simulink model "control_system"  (R2024a)
settings: Solver=VariableStepAuto  StartTime=0.0  StopTime=10.0  RelTol=1e-3
undefined symbols (not defined in the file): a, Cvx1, Cvx2, Cwy1, Cwy2, Jy, K, k, K1_k, K1_m, K2, K2_m, L11, L55, m, Mb, T, Umax, V_streem
libraries: dspsnks4 x1
settings Model: Creator=gbogu  LastModifiedBy=mikle
settings RTWCC: GPUComputeCapability=3.5

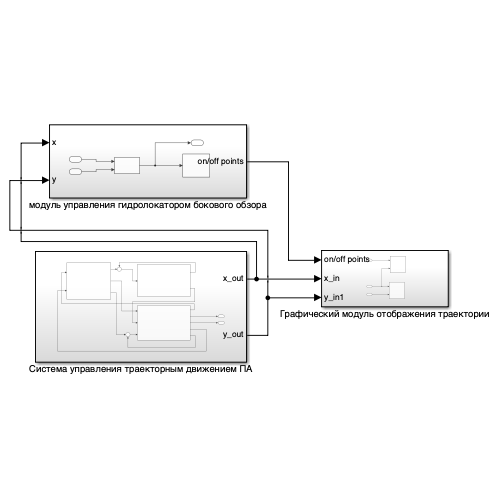
[thumbnail: Simulink's stored preview of the top-level diagram]
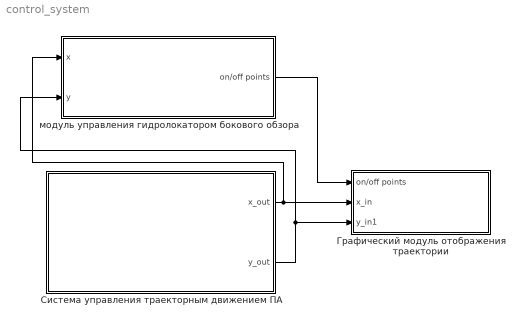
== system control_system ==
  Графический модуль отображения траектории : Subsystem
  Система управления траекторным движением ПА : Subsystem
  модуль управления гидролокатором бокового обзора : Subsystem
  wires:
  Система управления траекторным движением ПА/1(x_out) -> модуль управления гидролокатором бокового обзора/1(x), Графический модуль отображения траектории/2(x_in)
  Система управления траекторным движением ПА/2(y_out) -> модуль управления гидролокатором бокового обзора/2(y), Графический модуль отображения траектории/3(y_in1)
  модуль управления гидролокатором бокового обзора/1(on/off points) -> Графический модуль отображения траектории/1(on/off points)

== system control_system/Графический модуль отображения траектории ==
  on/off points : Inport
  x_in : Inport  Port=2
  y_in1 : Inport  Port=3
  XY Graph : Record  FileSettingsInternal="{\"entries\":[{\"content\":{\"excelSettings\":{\"content\":{},\"type\":\"Streamout.ExcelSettings\"}},\"type\":\"Streamout.FileSettingStorage\",\"uuid\":\"\"}],\"packageUris\":[\"http:\\/\\/schema.mathworks.com\\/mf0\\/streamout_blocks\\/R2020a\"],\"version\":\"1.0\"}"  Layout=[1 1]  SignalsInternal="{\"entries\":[{\"content\":{\"signals\":[{\"content\":{\"blockPath\":[],\"dimensions\":[1],\"domain\":\"\",\"lineColor\":\"#a2142f\",\"plots\":[ 1 ],\"port\":1,\"signalID\":1,\"signalName\":\"XY Graph:1\"},\"type\":\"RecordBlkView.Signal\",\"uuid\":\"\"},{\"content\":{\"blockPath\":[],\"dimensions\":[1],\"domain\":\"\",\"lineColor\":\"#139fff\",\"plots\":[ 1 ],\"port\":2,\"signalID\":2,\"signalName\":\"XY Graph:2\"},\"type\":\"RecordBlkView.Signal\",\"uuid\":\"\"}]},\"type\":\"RecordBlkView.InputSignals\",\"uuid\":\"\"}],\"packageUris\":[\"http:\\/\\/schema.mathworks.com\\/mf0\\/streamout_blocks\\/R2020a\"],\"version\":\"1.0\"}"  VisualizationBindings="{\"xyplotplugin\":{\"info\":[{\"series\":[{\"bindingParametersList\":[{\"parameter\":\"X-Axis\",\"signalID\":1,\"signalName\":\"XY Graph:1\"},{\"parameter\":\"Y-Axis\",\"signalID\":2,\"signalName\":\"XY Graph:2\"}],\"seriesID\":0}],\"subplotID\":1}]}}"  CompatibilityTag=XY
  XY Graph1 : Record  FileSettingsInternal="{\"entries\":[{\"content\":{\"excelSettings\":{\"content\":{},\"type\":\"Streamout.ExcelSettings\"}},\"type\":\"Streamout.FileSettingStorage\",\"uuid\":\"\"}],\"packageUris\":[\"http:\\/\\/schema.mathworks.com\\/mf0\\/streamout_blocks\\/R2020a\"],\"version\":\"1.0\"}"  Layout=[1 1]  SignalsInternal="{\"entries\":[{\"content\":{\"signals\":[{\"content\":{\"blockPath\":[],\"dimensions\":[1],\"domain\":\"\",\"lineColor\":\"#a2142f\",\"plots\":[ 1 ],\"port\":1,\"signalID\":1,\"signalName\":\"XY Graph:1\"},\"type\":\"RecordBlkView.Signal\",\"uuid\":\"\"},{\"content\":{\"blockPath\":[],\"dimensions\":[1],\"domain\":\"\",\"lineColor\":\"#139fff\",\"plots\":[ 1 ],\"port\":2,\"signalID\":2,\"signalName\":\"XY Graph:2\"},\"type\":\"RecordBlkView.Signal\",\"uuid\":\"\"}]},\"type\":\"RecordBlkView.InputSignals\",\"uuid\":\"\"}],\"packageUris\":[\"http:\\/\\/schema.mathworks.com\\/mf0\\/streamout_blocks\\/R2020a\"],\"version\":\"1.0\"}"  VisualizationBindings="{\"xyplotplugin\":{\"info\":[{\"series\":[{\"bindingParametersList\":[{\"parameter\":\"X-Axis\",\"signalID\":1,\"signalName\":\"XY Graph:1\"},{\"parameter\":\"Y-Axis\",\"signalID\":2,\"signalName\":\"XY Graph:2\"}],\"seriesID\":0}],\"subplotID\":1}]}}"  CompatibilityTag=XY
  wires:
  y_in1/1 -> XY Graph/2  "y"
  x_in/1 -> XY Graph1/2, XY Graph/1  "r_in"
  on/off points/1 -> XY Graph1/1

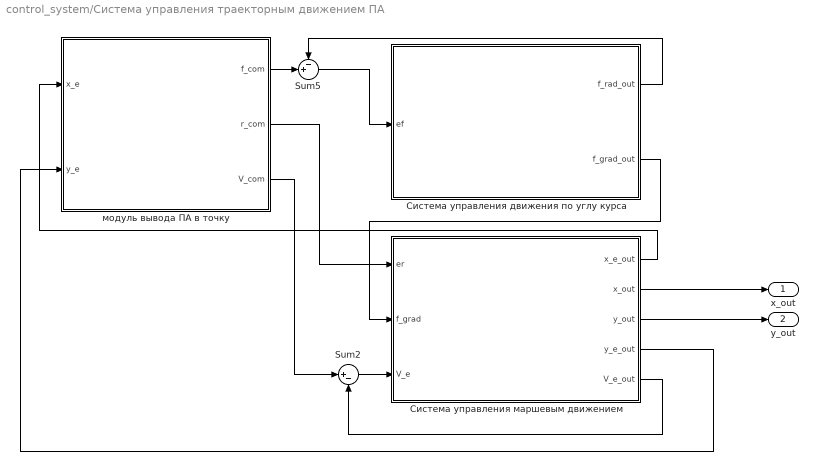
== system control_system/Система управления траекторным движением ПА ==
  Sum2 : Sum  Inputs=|+-
  Sum5 : Sum  Inputs=-+|
  "Система управления движения по углу курса " : Subsystem
  Система управления маршевым движением : Subsystem
  модуль вывода ПА в точку : Subsystem
  x_out : Outport
  y_out : Outport  Port=2
  wires:
  модуль вывода ПА в точку/1(f_com) -> Sum5/2
  модуль вывода ПА в точку/3(V_com) -> Sum2/1
  модуль вывода ПА в точку/2(r_com) -> Система управления маршевым движением/1(er)
  Sum2/1 -> Система управления маршевым движением/3(V_e)
  Система управления маршевым движением/1(x_e_out) -> модуль вывода ПА в точку/1(x_e)
  Система управления маршевым движением/2(x_out) -> x_out/1
  Система управления маршевым движением/3(y_out) -> y_out/1
  Система управления маршевым движением/4(y_e_out) -> модуль вывода ПА в точку/2(y_e)
  Система управления маршевым движением/5(V_e_out) -> Sum2/2
  "Система управления движения по углу курса "/2(f_grad_out) -> Система управления маршевым движением/2(f_grad)
  Sum5/1 -> "Система управления движения по углу курса "/1(ef)
  "Система управления движения по углу курса "/1(f_rad_out) -> Sum5/1

== system control_system/модуль управления гидролокатором бокового обзора ==
  x : Inport
  y : Inport  Port=2
  Function Caller : FunctionCaller  FunctionPrototype=y = f(x,y)  InputArgumentSpecifications=<Enter example>  OutputArgumentSpecifications=<Enter example>
  гидролокатор бокового обзора : dspsnks4/Audio Device Writer  Driver=CoreAudio  Device=Default  InheritSampleRate=on  SampleRate=44100  BitDepth=16-bit integer  BufferSize=4096  NumBuffers=10  DefaultOutputChannelMapping=on  OutputChannelMapping=1:2  OutputNumUnderrunSamples=off  DriverIdx=5  DeviceWarnFlag=''
  on/off points : Outport
  wires:
  x/1 -> Function Caller/1
  y/1 -> Function Caller/2
  Function Caller/1 -> on/off points/1, гидролокатор бокового обзора/1

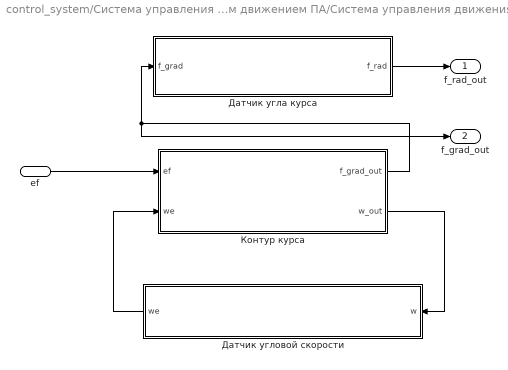
== system control_system/Система управления траекторным движением ПА/Система управления движения по углу курса  ==
  ef : Inport
  Датчик угла курса : Subsystem
  Датчик угловой скорости : Subsystem
  Контур курса : Subsystem
  f_rad_out : Outport
  f_grad_out : Outport  Port=2
  wires:
  ef/1 -> Контур курса/1(ef)
  Контур курса/2(w_out) -> Датчик угловой скорости/1(w)
  Контур курса/1(f_grad_out) -> f_grad_out/1, Датчик угла курса/1(f_grad)
  Датчик угла курса/1(f_rad) -> f_rad_out/1
  Датчик угловой скорости/1(we) -> Контур курса/2(we)

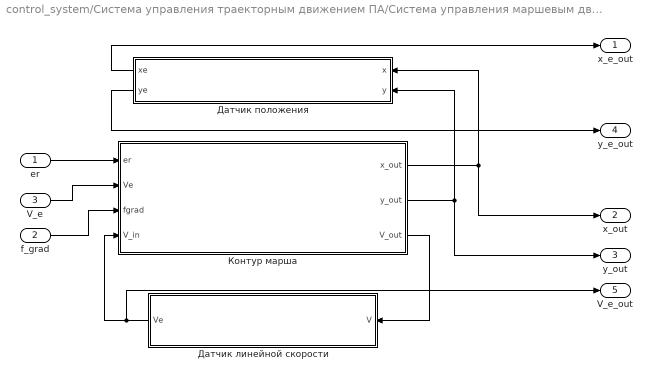
== system control_system/Система управления траекторным движением ПА/Система управления маршевым движением ==
  er : Inport
  f_grad : Inport  Port=2
  V_e : Inport  Port=3
  Датчик линейной скорости : Subsystem
  Датчик положения : Subsystem
  Контур марша : Subsystem
  x_e_out : Outport
  x_out : Outport  Port=2
  y_out : Outport  Port=3
  y_e_out : Outport  Port=4
  V_e_out : Outport  Port=5
  wires:
  er/1 -> Контур марша/1(er)
  Датчик положения/2(ye) -> y_e_out/1
  Датчик положения/1(xe) -> x_e_out/1
  Контур марша/3(V_out) -> Датчик линейной скорости/1(V)
  V_e/1 -> Контур марша/2(Ve)
  Контур марша/1(x_out) -> Датчик положения/1(x), x_out/1
  Контур марша/2(y_out) -> Датчик положения/2(y), y_out/1
  f_grad/1 -> Контур марша/3(fgrad)
  Датчик линейной скорости/1(Ve) -> Контур марша/4(V_in), V_e_out/1

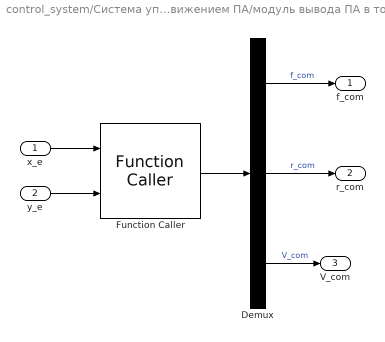
== system control_system/Система управления траекторным движением ПА/модуль вывода ПА в точку ==
  x_e : Inport
  y_e : Inport  Port=2
  Demux : Demux  Outputs=3
  Function Caller : FunctionCaller  FunctionPrototype=Vel = f(x_e,y_e)  InputArgumentSpecifications=<Enter example>  OutputArgumentSpecifications=<Enter example>
  f_com : Outport
  r_com : Outport  Port=2
  V_com : Outport  Port=3
  wires:
  Demux/3 -> V_com/1  "V_com"
  Demux/1 -> f_com/1  "f_com"
  Demux/2 -> r_com/1  "r_com"
  y_e/1 -> Function Caller/2
  x_e/1 -> Function Caller/1
  Function Caller/1 -> Demux/1

== system control_system/Система управления траекторным движением ПА/Система управления движения по углу курса /Датчик угла курса ==
  f_grad : Inport
  Gain10 : Gain  Gain=pi/180
  angle sensore : Gain  Gain=93.1395
  f_rad : Outport
  wires:
  Gain10/1 -> f_rad/1  "frad"
  f_grad/1 -> angle sensore/1
  angle sensore/1 -> Gain10/1  "fe"

== system control_system/Система управления траекторным движением ПА/Система управления движения по углу курса /Датчик угловой скорости ==
  w : Inport
  omega sensor : Gain  Gain=93.1395
  we : Outport
  wires:
  omega sensor/1 -> we/1  "we"
  w/1 -> omega sensor/1

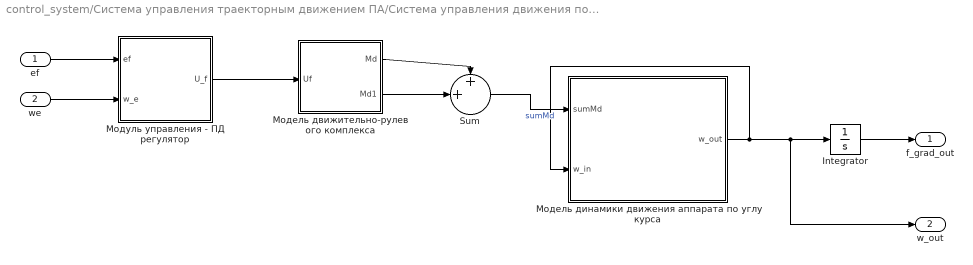
== system control_system/Система управления траекторным движением ПА/Система управления движения по углу курса /Контур курса ==
  ef : Inport
  we : Inport  Port=2
  Integrator : Integrator
  Sum : Sum  Inputs=++|
  Модель движительно-рулевого комплекса : Subsystem
  Модель динамики движения аппарата по углу курса : Subsystem
  Модуль управления - ПД регулятор : Subsystem
  f_grad_out : Outport
  w_out : Outport  Port=2
  wires:
  Модель динамики движения аппарата по углу курса/1(w_out) -> Модель динамики движения аппарата по углу курса/2(w_in), w_out/1, Integrator/1
  ef/1 -> Модуль управления - ПД регулятор/1(ef)
  we/1 -> Модуль управления - ПД регулятор/2(w_e)
  Модель движительно-рулевого комплекса/1(Md) -> Sum/1
  Sum/1 -> Модель динамики движения аппарата по углу курса/1(sumMd)  "sumMd"
  Модуль управления - ПД регулятор/1(U_f) -> Модель движительно-рулевого комплекса/1(Uf)
  Модель движительно-рулевого комплекса/2(Md1) -> Sum/2
  Integrator/1 -> f_grad_out/1

== system control_system/Система управления траекторным движением ПА/Система управления маршевым движением/Датчик линейной скорости ==
  V : Inport
  speed sensor : Gain  Gain=93.1395
  Ve : Outport
  wires:
  V/1 -> speed sensor/1
  speed sensor/1 -> Ve/1  "we"

== system control_system/Система управления траекторным движением ПА/Система управления маршевым движением/Датчик положения ==
  x : Inport
  y : Inport  Port=2
  position sensore : Gain  Gain=93.1395
  position sensore1 : Gain  Gain=93.1395
  xe : Outport
  ye : Outport  Port=2
  wires:
  x/1 -> position sensore/1
  y/1 -> position sensore1/1
  position sensore1/1 -> ye/1  "fe"
  position sensore/1 -> xe/1  "fe"

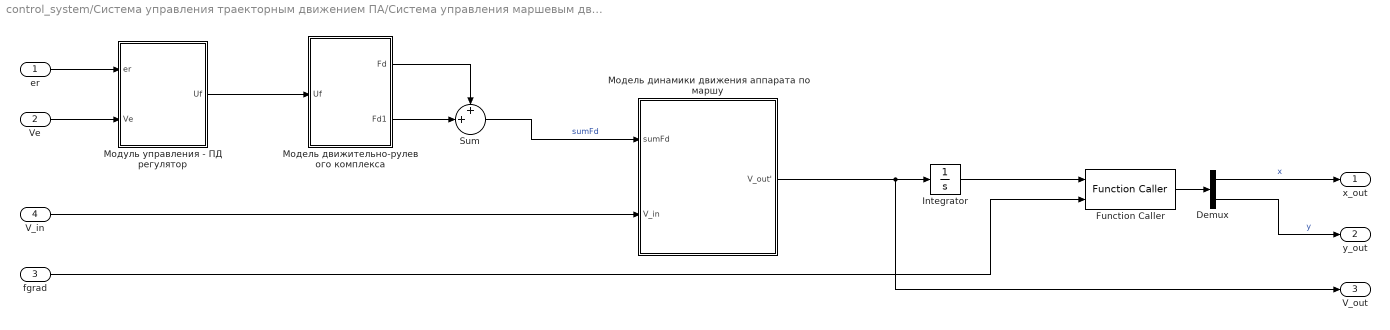
== system control_system/Система управления траекторным движением ПА/Система управления маршевым движением/Контур марша ==
  er : Inport
  Ve : Inport  Port=2
  fgrad : Inport  Port=3
  V_in : Inport  Port=4
  Demux : Demux  Outputs=2
  Function Caller : FunctionCaller  FunctionPrototype=y = f(r_in,fgrad)  InputArgumentSpecifications=<Enter example>  OutputArgumentSpecifications=<Enter example>
  Integrator : Integrator
  Sum : Sum  Inputs=++|
  Модель движительно-рулевого комплекса : Subsystem
  Модель динамики движения аппарата по маршу : Subsystem
  Модуль управления - ПД регулятор : Subsystem
  x_out : Outport
  y_out : Outport  Port=2
  V_out : Outport  Port=3
  wires:
  Модель движительно-рулевого комплекса/2(Fd1) -> Sum/2
  V_in/1 -> Модель динамики движения аппарата по маршу/2(V_in)
  Модуль управления - ПД регулятор/1(Uf) -> Модель движительно-рулевого комплекса/1(Uf)
  Sum/1 -> Модель динамики движения аппарата по маршу/1(sumFd)  "sumFd"
  Модель движительно-рулевого комплекса/1(Fd) -> Sum/1
  Ve/1 -> Модуль управления - ПД регулятор/2(Ve)
  er/1 -> Модуль управления - ПД регулятор/1(er)
  Модель динамики движения аппарата по маршу/1(V_out') -> V_out/1, Integrator/1
  Function Caller/1 -> Demux/1
  Integrator/1 -> Function Caller/1
  fgrad/1 -> Function Caller/2
  Demux/1 -> x_out/1  "x"
  Demux/2 -> y_out/1  "y"

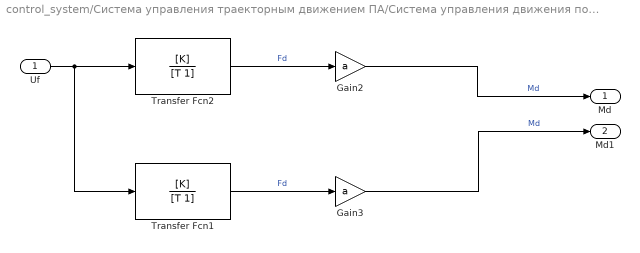
== system control_system/Система управления траекторным движением ПА/Система управления движения по углу курса /Контур курса/Модель движительно-рулевого комплекса ==
  Uf : Inport
  Gain2 : Gain  Gain=a
  Gain3 : Gain  Gain=a
  Transfer Fcn1 : TransferFcn  Numerator=[K]  Denominator=[T 1]
  Transfer Fcn2 : TransferFcn  Numerator=[K]  Denominator=[T 1]
  Md : Outport
  Md1 : Outport  Port=2
  wires:
  Gain3/1 -> Md1/1  "Md"
  Gain2/1 -> Md/1  "Md"
  Uf/1 -> Transfer Fcn1/1, Transfer Fcn2/1
  Transfer Fcn2/1 -> Gain2/1  "Fd"
  Transfer Fcn1/1 -> Gain3/1  "Fd"

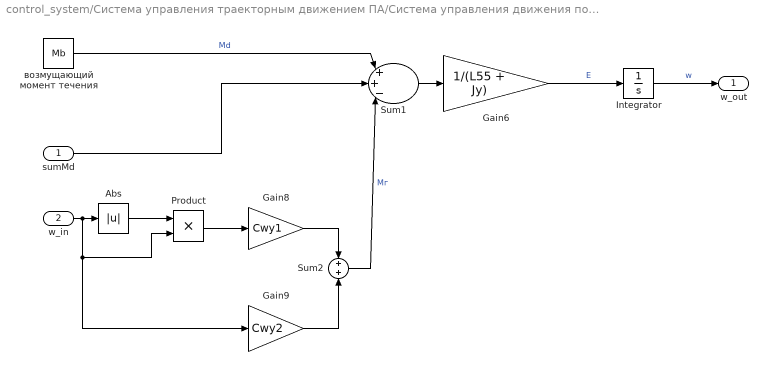
== system control_system/Система управления траекторным движением ПА/Система управления движения по углу курса /Контур курса/Модель динамики движения аппарата по углу курса ==
  sumMd : Inport
  w_in : Inport  Port=2
  Abs : Abs  SaturateOnIntegerOverflow=off
  Gain6 : Gain  Gain=1/(L55 + Jy)
  Gain8 : Gain  Gain=Cwy1
  Gain9 : Gain  Gain=Cwy2
  Integrator : Integrator
  Product : Product
  Sum1 : Sum  Inputs=|++-|
  Sum2 : Sum  Inputs=+|+
  возмущающий момент течения : Constant  Value=Mb
  w_out : Outport
  wires:
  Gain8/1 -> Sum2/1
  Sum1/1 -> Gain6/1
  Integrator/1 -> w_out/1  "w"
  Gain6/1 -> Integrator/1  "E"
  Sum2/1 -> Sum1/3  "Mг"
  w_in/1 -> Gain9/1, Product/2, Abs/1
  Gain9/1 -> Sum2/2
  sumMd/1 -> Sum1/2
  возмущающий момент течения/1 -> Sum1/1  "Md"
  Product/1 -> Gain8/1
  Abs/1 -> Product/1

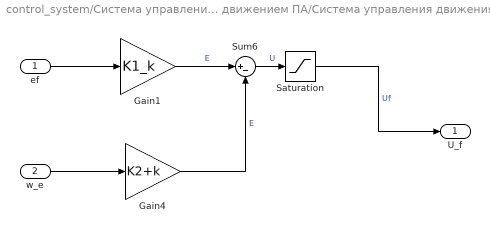
== system control_system/Система управления траекторным движением ПА/Система управления движения по углу курса /Контур курса/Модуль управления - ПД регулятор ==
  ef : Inport
  w_e : Inport  Port=2
  Gain1 : Gain  Gain=K1_k
  Gain4 : Gain  Gain=K2+k
  Saturation : Saturate  UpperLimit=Umax  LowerLimit=-Umax
  Sum6 : Sum  Inputs=|+-
  U_f : Outport
  wires:
  Sum6/1 -> Saturation/1  "U"
  ef/1 -> Gain1/1
  Gain4/1 -> Sum6/2  "E"
  Gain1/1 -> Sum6/1  "E"
  Saturation/1 -> U_f/1  "Uf"
  w_e/1 -> Gain4/1

== system control_system/Система управления траекторным движением ПА/Система управления маршевым движением/Контур марша/Модель движительно-рулевого комплекса ==
  Uf : Inport
  Transfer Fcn1 : TransferFcn  Numerator=[K]  Denominator=[T 1]
  Transfer Fcn2 : TransferFcn  Numerator=[K]  Denominator=[T 1]
  Fd : Outport
  Fd1 : Outport  Port=2
  wires:
  Transfer Fcn1/1 -> Fd1/1  "Fd"
  Uf/1 -> Transfer Fcn2/1, Transfer Fcn1/1
  Transfer Fcn2/1 -> Fd/1  "Fd"

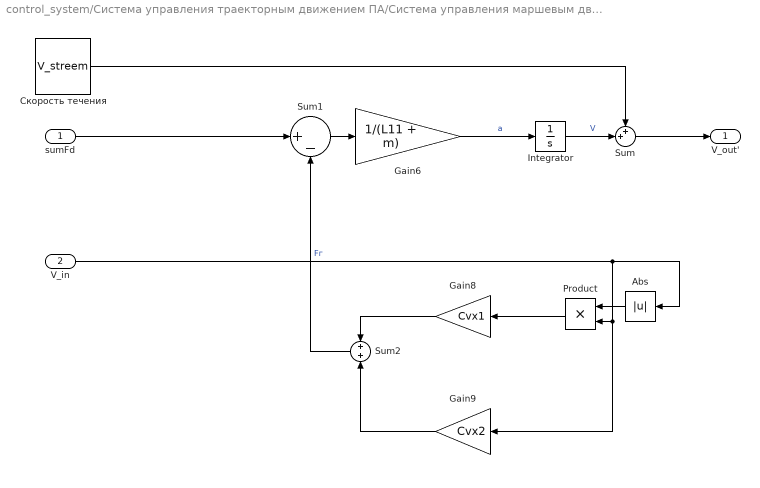
== system control_system/Система управления траекторным движением ПА/Система управления маршевым движением/Контур марша/Модель динамики движения аппарата по маршу ==
  sumFd : Inport
  V_in : Inport  Port=2
  Abs : Abs  SaturateOnIntegerOverflow=off
  Gain6 : Gain  Gain=1/(L11 + m)
  Gain8 : Gain  Gain=Cvx1
  Gain9 : Gain  Gain=Cvx2
  Integrator : Integrator
  Product : Product
  Sum : Sum  Inputs=++|
  Sum1 : Sum  Inputs=|+-
  Sum2 : Sum
  Скорость течения : Constant  Value=V_streem
  V_out' : Outport
  wires:
  Abs/1 -> Product/1
  Product/1 -> Gain8/1
  Gain9/1 -> Sum2/2
  Gain6/1 -> Integrator/1  "a"
  V_in/1 -> Abs/1, Gain9/1, Product/2
  Sum1/1 -> Gain6/1
  Gain8/1 -> Sum2/1
  Sum2/1 -> Sum1/2  "Fг"
  sumFd/1 -> Sum1/1
  Integrator/1 -> Sum/2  "V"
  Sum/1 -> V_out'/1
  Скорость течения/1 -> Sum/1

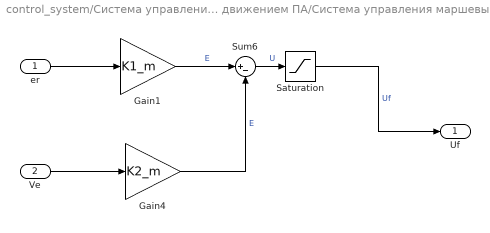
== system control_system/Система управления траекторным движением ПА/Система управления маршевым движением/Контур марша/Модуль управления - ПД регулятор ==
  er : Inport
  Ve : Inport  Port=2
  Gain1 : Gain  Gain=K1_m
  Gain4 : Gain  Gain=K2_m
  Saturation : Saturate  UpperLimit=Umax  LowerLimit=-Umax
  Sum6 : Sum  Inputs=|+-
  Uf : Outport
  wires:
  Ve/1 -> Gain4/1
  Saturation/1 -> Uf/1  "Uf"
  Gain1/1 -> Sum6/1  "E"
  Gain4/1 -> Sum6/2  "E"
  er/1 -> Gain1/1
  Sum6/1 -> Saturation/1  "U"
